simulink model "SimulinkTaskModuleAIL"  (Simulink 7.5)
settings: Solver=VariableStepDiscrete  StartTime=0.0  StopTime=100000  MaxStep=1  RelTol=1e-3
libraries: simulink x1
Description:
  | % Copyright (C) 2012 Nicholas K. Lincoln, Sandor M. Veres, Louise Dennis,
  | % Michael Fisher, and Alexei Lisitsa.
  | %
  | % This file is part of the EASS (Engineering Autonomous Space Software)
  | % Demonstrator Set.
  | %
  | % The EASS Demonstrator Set is free software: you can redistribute it
  | % and/or modify it under the terms of the GNU Lesser General Public License
  | % as published by the Free Software Foundation, either version 3 of the
  | % License, or (at your option) any later version.
  | %
  | % The EASS Demonstrator Set is distributed in the hope that it will be
  | % useful, but WITHOUT ANY WARRANTY; without even the implied warranty of
  | % MERCHANTABILITY or FITNESS FOR A PARTICULAR PURPOSE.  See the GNU Lesser
  | % General Public License for more details.
  | %
  | % You should have received a copy of the GNU Lesser General Public License
  | % along with the EASS Demonstrator Set.  If not, see
  | % <http://www.gnu.org/licenses/>.
settings Model: Creator=N K Lincoln  LastModifiedBy=lad
settings OptimizationCC: InitFltsAndDblsToZero=on
settings DebuggingCC: SaveWithParameterizedLinksMsg=none  SignalResolutionControl=TryResolveAllWithWarning  StrictBusMsg=Warning
settings GRTTargetCC: TargetFcnLib=ansi_tfl_tmw.mat

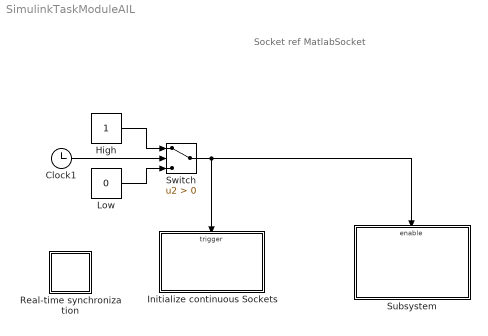
== system SimulinkTaskModuleAIL ==
  note: Socket ref MatlabSocket
  Clock1 : Clock
      settings: Decimation=10
  High : Constant  OutDataType=sfix(16)  OutScaling=2^0
  Initialize continuous Sockets : Subsystem  TreatAsAtomicUnit=on
  Low : Constant  Value=0  OutDataType=sfix(16)  OutScaling=2^0
  Real-time synchronization : Subsystem
  Subsystem : Subsystem
  Switch : Switch  Criteria=u2 > Threshold
  wires:
  Low/1 -> Switch/3
  High/1 -> Switch/1
  Clock1/1 -> Switch/2
  Switch/1 -> Initialize continuous Sockets/Trigger, Subsystem/Enable

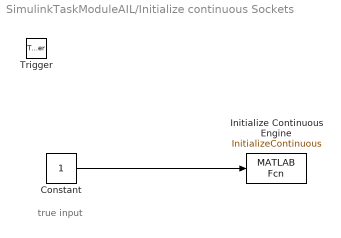
== system SimulinkTaskModuleAIL/Initialize continuous Sockets ==
  note: true input
  Trigger : TriggerPort
  Constant : Constant  OutDataType=fixdt(1, 16)  OutScaling=2^0
  Initialize Continuous Engine : MATLABFcn  MATLABFcn=InitializeContinuous  OutputDimensions=0
  wires:
  Constant/1 -> Initialize Continuous Engine/1

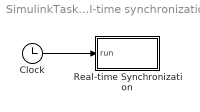
== system SimulinkTaskModuleAIL/Real-time synchronization ==
  Clock : Clock
      settings: Decimation=10
  Real-time Synchronization : Subsystem
  wires:
  Clock/1 -> Real-time Synchronization/1(run)

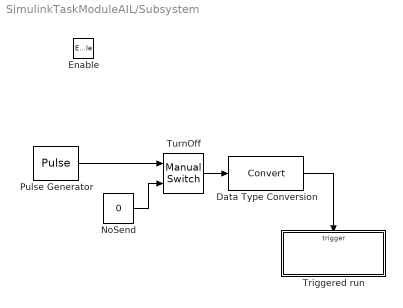
== system SimulinkTaskModuleAIL/Subsystem ==
  Enable : EnablePort
  Data Type Conversion : DataTypeConversion  OutDataType=sfix(16)  OutScaling=2^0
  NoSend : Constant  Value=0  OutDataType=sfix(16)  OutScaling=2^0
  Pulse Generator : DiscretePulseGenerator  PulseType=Time based  Amplitude=1  Period=0.001  PulseWidth=50  PhaseDelay=0  SampleTime=1
  Triggered run : Subsystem  TreatAsAtomicUnit=on
  TurnOff : simulink/Signal Routing/Manual Switch  SystemSampleTime=-1  sw=1  action=0  varsize=off
  wires:
  Data Type Conversion/1 -> Triggered run/Trigger
  NoSend/1 -> TurnOff/2
  Pulse Generator/1 -> TurnOff/1
  TurnOff/1 -> Data Type Conversion/1

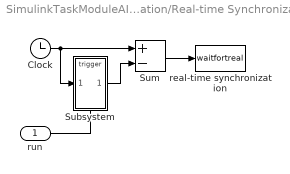
== system SimulinkTaskModuleAIL/Real-time synchronization/Real-time Synchronization ==
  run : Inport
  Clock : Clock
      settings: Decimation=10
  Subsystem : Subsystem  TreatAsAtomicUnit=on
  Sum : Sum  Inputs=+-  SaturateOnIntegerOverflow=on  InputSameDT=on  OutDataTypeStr=Inherit: Same as first input
  real-time synchronization : MATLABFcn  MATLABFcn=waitfortreal  OutputDimensions=0
  wires:
  run/1 -> Subsystem/Trigger
  Sum/1 -> real-time synchronization/1
  Subsystem/1(Out) -> Sum/2
  Clock/1 -> Sum/1, Subsystem/1(In)

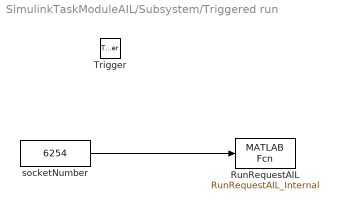
== system SimulinkTaskModuleAIL/Subsystem/Triggered run ==
  Trigger : TriggerPort
  RunRequestAIL : MATLABFcn  MATLABFcn=RunRequestAIL_Internal  OutputDimensions=0
  socketNumber : Constant  Value=6254  OutDataType=sfix(16)  OutScaling=2^0
  wires:
  socketNumber/1 -> RunRequestAIL/1

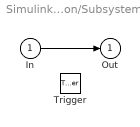
== system SimulinkTaskModuleAIL/Real-time synchronization/Real-time Synchronization/Subsystem ==
  In : Inport
  Trigger : TriggerPort
  Out : Outport  InitialOutput=0
  wires:
  In/1 -> Out/1
